simulink model "Hiv_med_maalestoy"  (R2023b)
settings: Solver=VariableStepAuto  StartTime=0.0  StopTime=10.0  RelTol=1e-3
values from neighbouring files (symbols this model uses):
  D_hiv_fart = [M(3),rho_vann*Cd*A_z*Z_2]    [Overforingsfunksjon_Translasjon.m]
libraries: simulink x1
settings Model: Creator=anneb  LastModifiedBy=anneb

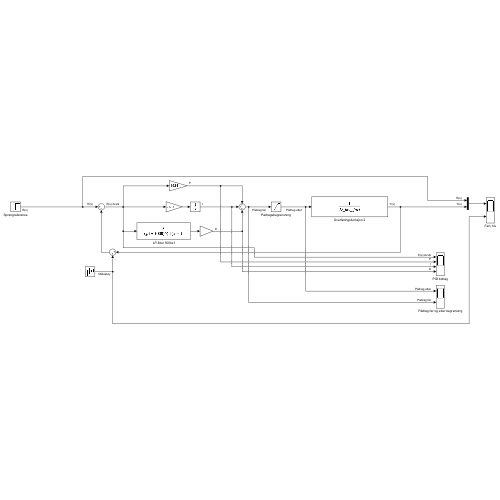
[thumbnail: Simulink's stored preview of the top-level diagram]
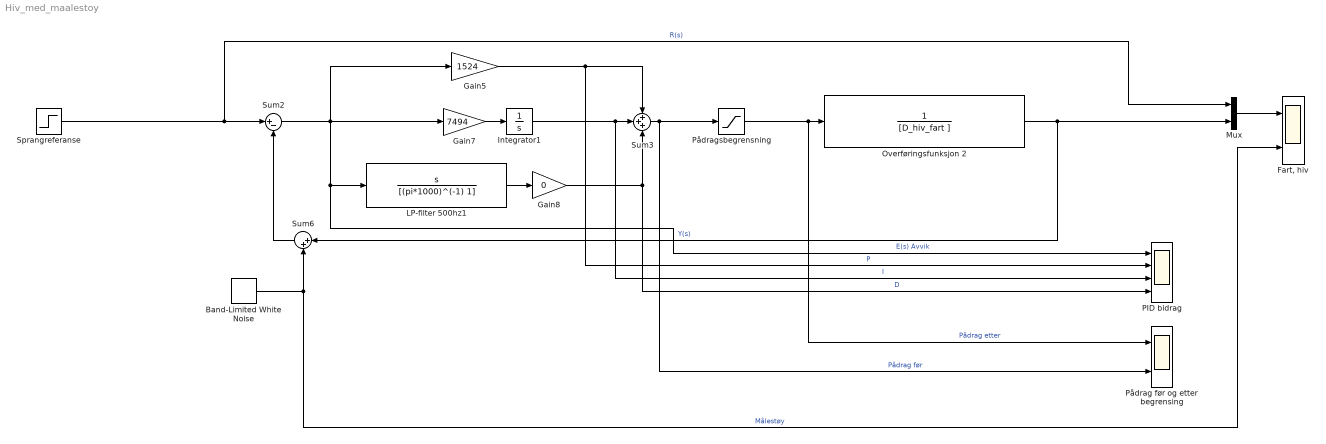
== system Hiv_med_maalestoy ==
  " LP-filter 500hz1" : TransferFcn  Numerator=[1 0]  Denominator=[(pi*1000)^(-1) 1]
  Band-Limited White Noise : simulink/Sources/Band-Limited White Noise  Cov=[0.000001]  Ts=0.1  seed=[23341]
  "Fart, hiv" : Scope  NumInputPorts=2
  Gain5 : Gain  Gain=1524
  Gain7 : Gain  Gain=7494
  Gain8 : Gain  Gain=0
  Integrator1 : Integrator
  Mux : Mux  Inputs=2
  Overføringsfunksjon 2 : TransferFcn  Denominator=[D_hiv_fart ]
  PID bidrag : Scope  NumInputPorts=4
  Pådrag før og etter begrensing : Scope  NumInputPorts=2
  Pådragsbegrensning : Saturate  UpperLimit=115  LowerLimit=-145
  Sprangreferanse : Step  After=0.0325  SampleTime=0
  Sum2 : Sum  Inputs=|+-
  Sum3 : Sum  Inputs=+++
  Sum6 : Sum  Inputs=|++
  wires:
  Sum6/1 -> Sum2/2
  Gain5/1 -> Sum3/1, PID bidrag/2  "P"
  Integrator1/1 -> PID bidrag/3, Sum3/2  "I"
  Overføringsfunksjon 2/1 -> Mux/2, Sum6/1  "Y(s)"
  Sprangreferanse/1 -> Mux/1, Sum2/1  "R(s)"
  " LP-filter 500hz1"/1 -> Gain8/1
  Sum3/1 -> Pådragsbegrensning/1, Pådrag før og etter begrensing/2  "Pådrag før"
  Gain7/1 -> Integrator1/1
  Gain8/1 -> Sum3/3, PID bidrag/4  "D"
  Band-Limited White Noise/1 -> Sum6/2, "Fart, hiv"/2  "Målestøy"
  Sum2/1 -> PID bidrag/1, " LP-filter 500hz1"/1, Gain7/1, Gain5/1  "E(s) Avvik"
  Pådragsbegrensning/1 -> Pådrag før og etter begrensing/1, Overføringsfunksjon 2/1  "Pådrag etter"
  Mux/1 -> "Fart, hiv"/1
